simulink model "quantization3"  (Simulink 8.3)
settings: Solver=ode45  StartTime=0.0  StopTime=20  RelTol=1e-3
libraries: simulink x2
settings Model: Creator=Liu Guopin  LastModifiedBy=Liu Guopin
settings OptimizationCC: ExpressionDepthLimit=2147483647
settings DebuggingCC: FcnCallInpInsideContextMsg=UseLocalSettings  StrictBusMsg=Warning

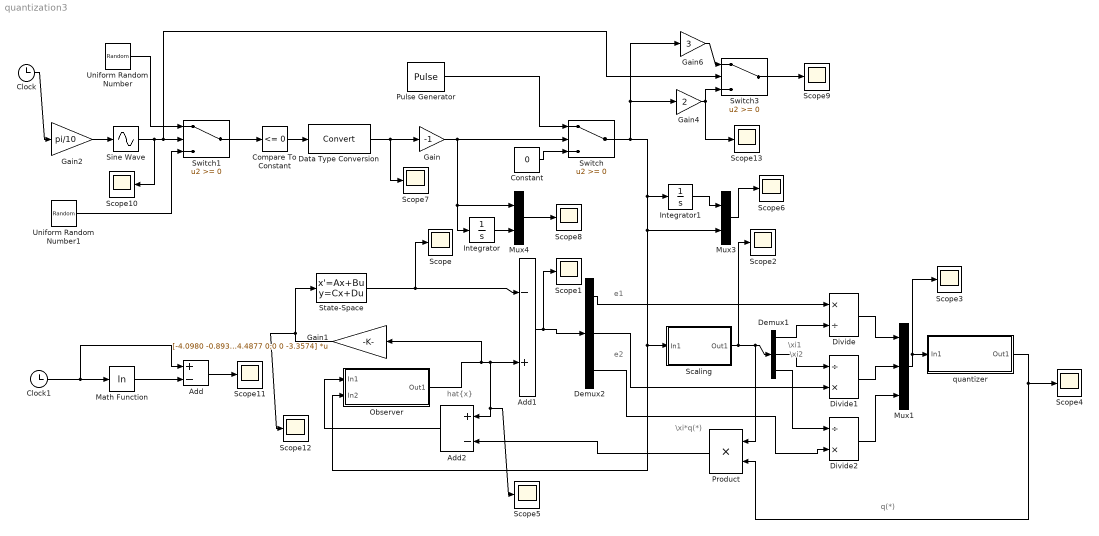
== system quantization3 ==
  note: e1
  note: e2
  note: \xi1
  note: \xi2
  note: hat{x}
  note: q(*)
  note: \xi*q(*)
  Add : Sum  Inputs=+-
  Add1 : Sum  Inputs=-+
  Add2 : Sum  Inputs=+-
  Clock : Clock
  Clock1 : Clock
  Compare To Constant : simulink/Logic and Bit Operations/Compare To Constant  relop=<=  const=0  OutDataTypeStr=boolean
  Constant : Constant  Value=0
  Data Type Conversion : DataTypeConversion
  Demux1 : Demux  Outputs=3
  Demux2 : Demux  Outputs=3
  Divide : Product  Inputs=*/
  Divide1 : Product  Inputs=/*
  Divide2 : Product  Inputs=/*
  Gain : Gain  Gain=-1
  Gain1 : Gain  Gain=[-4.0980 -0.8936 0; -0.8936 -4.4877 0;0 0 -3.3574]  Multiplication=Matrix(K*u) (u vector)
  Gain2 : Gain  Gain=pi/10
  Gain4 : Gain  Gain=2
  Gain6 : Gain  Gain=3
  Integrator : Integrator
  Integrator1 : Integrator
  Math Function : Math  Operator=log  SaturateOnIntegerOverflow=on
  Mux1 : Mux  Inputs=3
  Mux3 : Mux  Inputs=2
  Mux4 : Mux  Inputs=2
  Observer : Subsystem
  Product : Product  RndMeth=Zero
  Pulse Generator : DiscretePulseGenerator  PulseType=Time based  Period=0.1  PulseWidth=5
  Scaling : Subsystem
  Scope{,1..13} (14 alike) : Scope
      Scope1 settings: SaveName=ScopeData2
      Scope10 settings: SaveName=ScopeData11
      Scope11 settings: SaveName=ScopeData12
      Scope12 settings: SaveName=ScopeData15
      Scope13 settings: SaveName=ScopeData17
      Scope2 settings: SaveName=ScopeData3
      Scope3 settings: SaveName=ScopeData4
      Scope4 settings: SaveName=ScopeData5
      Scope5 settings: SaveName=ScopeData6
      Scope6 settings: SaveName=ScopeData7
      Scope7 settings: SaveName=ScopeData8
      Scope8 settings: SaveName=ScopeData9
      Scope9 settings: SaveName=ScopeData10
  Sine Wave : Sin  TimeSource=Use external signal  SampleTime=0
  State-Space : StateSpace  A=[2 1 0;0 2 0;0 0 1.5]  B=eye(3)  C=eye(3)  D=[0 0 0;0 0 0;0 0 0]  X0=[1.2;-0.8;0.5]
  Switch : Switch
  Switch1 : Switch
  Switch3 : Switch
  Uniform Random Number : UniformRandomNumber  Minimum=-1.37  Maximum=0.63  SampleTime=0.2
  Uniform Random Number1 : UniformRandomNumber  Minimum=-0.8  Maximum=1.2  SampleTime=0.2
  quantizer : Subsystem
  wires:
  Compare To Constant/1 -> Data Type Conversion/1
  Gain/1 -> Switch/2, Integrator/1, Mux4/1
  Data Type Conversion/1 -> Scope7/1, Gain/1
  State-Space/1 -> Add1/1, Scope/1
  Observer/1(Out1) -> Gain1/1, Add1/2, Add2/1, Scope5/1
  Gain1/1 -> State-Space/1, Scope12/1
  Scaling/1(Out1) -> Demux1/1, Product/1, Scope2/1
  Demux1/2 -> Divide1/1
  Demux1/1 -> Divide/2
  Demux2/1 -> Divide/1
  Demux2/2 -> Divide1/2
  Divide/1 -> Mux1/1
  Divide1/1 -> Mux1/2
  Mux1/1 -> quantizer/1(In1), Scope3/1
  quantizer/1(Out1) -> Product/2, Scope4/1
  Product/1 -> Add2/2
  Add2/1 -> Observer/1(In1)
  Constant/1 -> Switch/3
  Pulse Generator/1 -> Switch/1
  Switch/1 -> Integrator1/1, Scaling/1(In1), Observer/2(In2), Mux3/2, Gain6/1, Gain4/1
  Add1/1 -> Demux2/1, Scope1/1
  Clock/1 -> Gain2/1
  Gain2/1 -> Sine Wave/1
  Integrator1/1 -> Mux3/1
  Mux3/1 -> Scope6/1
  Integrator/1 -> Mux4/2
  Mux4/1 -> Scope8/1
  Sine Wave/1 -> Scope10/1, Switch1/2, Switch3/2
  Uniform Random Number1/1 -> Switch1/3
  Uniform Random Number/1 -> Switch1/1
  Switch1/1 -> Compare To Constant/1
  Clock1/1 -> Math Function/1, Add/1
  Math Function/1 -> Add/2
  Add/1 -> Scope11/1
  Demux1/3 -> Divide2/1
  Demux2/3 -> Divide2/2
  Divide2/1 -> Mux1/3
  Gain6/1 -> Switch3/1
  Gain4/1 -> Switch3/3, Scope13/1
  Switch3/1 -> Scope9/1

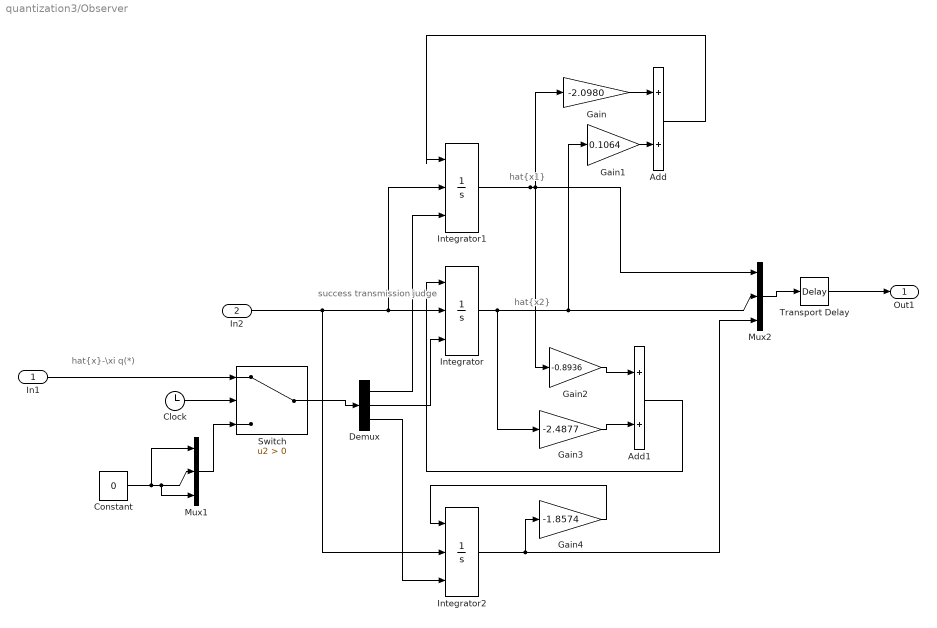
== system quantization3/Observer ==
  note: hat{x2}
  note: hat{x}-\xi q(*)
  note: success transmission judge
  note: hat{x1}
  In1 : Inport
  In2 : Inport  Port=2
  Add : Sum
  Add1 : Sum
  Clock : Clock
  Constant : Constant  Value=0
  Demux : Demux  Outputs=3
  Gain : Gain  Gain=-2.0980
  Gain1 : Gain  Gain=0.1064
  Gain2 : Gain  Gain=-0.8936
  Gain3 : Gain  Gain=-2.4877
  Gain4 : Gain  Gain=-1.8574
  Integrator : Integrator  ExternalReset=rising  InitialConditionSource=external
  Integrator1 : Integrator  ExternalReset=rising  InitialConditionSource=external
  Integrator2 : Integrator  ExternalReset=rising  InitialConditionSource=external
  Mux1 : Mux  Inputs=3
  Mux2 : Mux  Inputs=3
  Switch : Switch  Criteria=u2 > Threshold
  Transport Delay : TransportDelay  DelayTime=0.00000001
  Out1 : Outport
  wires:
  In1/1 -> Switch/1
  Clock/1 -> Switch/2
  Constant/1 -> Mux1/1, Mux1/2, Mux1/3
  Mux1/1 -> Switch/3
  Switch/1 -> Demux/1
  In2/1 -> Integrator/2, Integrator1/2, Integrator2/2
  Integrator/1 -> Mux2/2, Gain1/1, Gain3/1
  Demux/1 -> Integrator1/3
  Demux/2 -> Integrator/3
  Integrator1/1 -> Mux2/1, Gain/1, Gain2/1
  Gain1/1 -> Add/2
  Gain/1 -> Add/1
  Gain3/1 -> Add1/2
  Gain2/1 -> Add1/1
  Add/1 -> Integrator1/1
  Add1/1 -> Integrator/1
  Transport Delay/1 -> Out1/1
  Demux/3 -> Integrator2/3
  Mux2/1 -> Transport Delay/1
  Integrator2/1 -> Mux2/3, Gain4/1
  Gain4/1 -> Integrator2/1

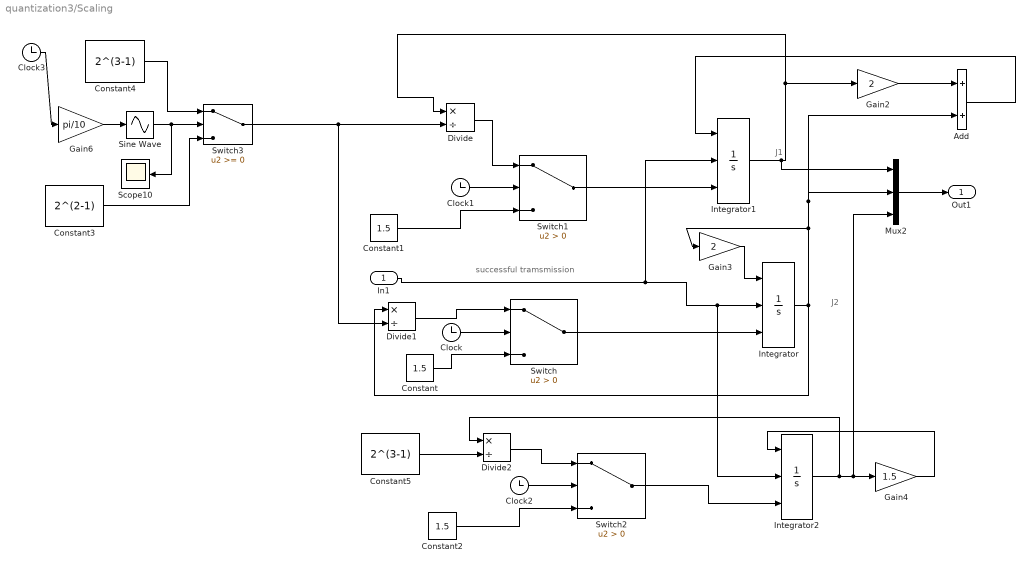
== system quantization3/Scaling ==
  note: J1
  note: J2
  note: successful tramsmission
  In1 : Inport
  Add : Sum
  Clock{,1..3} (4 alike) : Clock
  Constant : Constant  Value=1.5
  Constant1 : Constant  Value=1.5
  Constant2 : Constant  Value=1.5
  Constant3 : Constant  Value=2^(2-1)
  Constant4 : Constant  Value=2^(3-1)
  Constant5 : Constant  Value=2^(3-1)
  Divide : Product  Inputs=*/
  Divide1 : Product  Inputs=*/
  Divide2 : Product  Inputs=*/
  Gain2 : Gain  Gain=2
  Gain3 : Gain  Gain=2
  Gain4 : Gain  Gain=1.5
  Gain6 : Gain  Gain=pi/10
  Integrator : Integrator  ExternalReset=rising  InitialConditionSource=external
  Integrator1 : Integrator  ExternalReset=rising  InitialConditionSource=external
  Integrator2 : Integrator  ExternalReset=rising  InitialConditionSource=external
  Mux2 : Mux  Inputs=3
  Scope10 : Scope
      settings: SaveName=ScopeData14
  Sine Wave : Sin  TimeSource=Use external signal  SampleTime=0
  Switch : Switch  Criteria=u2 > Threshold
  Switch1 : Switch  Criteria=u2 > Threshold
  Switch2 : Switch  Criteria=u2 > Threshold
  Switch3 : Switch
  Out1 : Outport
  wires:
  Clock/1 -> Switch/2
  Constant/1 -> Switch/3
  Clock1/1 -> Switch1/2
  Constant1/1 -> Switch1/3
  Switch/1 -> Integrator/3
  Switch1/1 -> Integrator1/3
  In1/1 -> Integrator1/2, Integrator/2, Integrator2/2
  Integrator1/1 -> Gain2/1, Divide/1, Mux2/1
  Integrator/1 -> Add/2, Mux2/2, Gain3/1, Divide1/1
  Add/1 -> Integrator1/1
  Mux2/1 -> Out1/1
  Gain2/1 -> Add/1
  Gain3/1 -> Integrator/1
  Clock2/1 -> Switch2/2
  Constant2/1 -> Switch2/3
  Integrator2/1 -> Gain4/1, Mux2/3, Divide2/1
  Switch2/1 -> Integrator2/3
  Gain4/1 -> Integrator2/1
  Divide2/1 -> Switch2/1
  Clock3/1 -> Gain6/1
  Gain6/1 -> Sine Wave/1
  Sine Wave/1 -> Switch3/2, Scope10/1
  Constant3/1 -> Switch3/3
  Constant4/1 -> Switch3/1
  Divide/1 -> Switch1/1
  Switch3/1 -> Divide/2, Divide1/2
  Divide1/1 -> Switch/1
  Constant5/1 -> Divide2/2

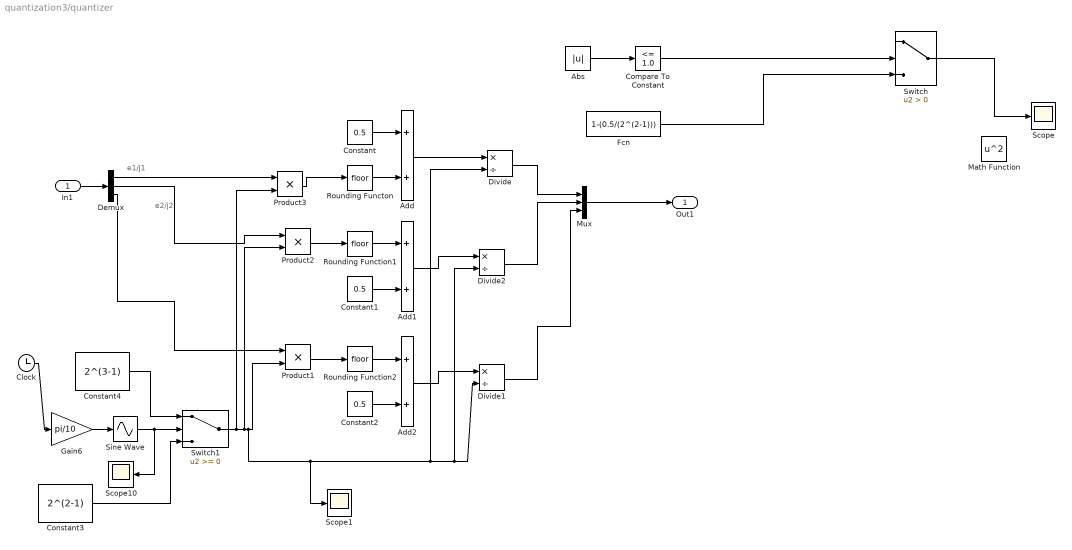
== system quantization3/quantizer ==
  note: e1/j1
  note: e2/j2
  In1 : Inport
  Abs : Abs
  Add : Sum
  Add1 : Sum
  Add2 : Sum
  Clock : Clock
  Compare To Constant : simulink/Logic and Bit Operations/Compare To Constant  SystemSampleTime=-1  relop=<=  const=1.0  LogicOutDataTypeMode=uint8  ZeroCross=off
  Constant : Constant  Value=0.5
  Constant1 : Constant  Value=0.5
  Constant2 : Constant  Value=0.5
  Constant3 : Constant  Value=2^(2-1)
  Constant4 : Constant  Value=2^(3-1)
  Demux : Demux  Outputs=3
  Divide : Product  Inputs=*/
  Divide1 : Product  Inputs=*/
  Divide2 : Product  Inputs=*/
  Fcn : Fcn  Expr=1-(0.5/(2^(2-1)))
  Gain6 : Gain  Gain=pi/10
  Math Function : Math  Operator=square  SaturateOnIntegerOverflow=on
  Mux : Mux  Inputs=3
  Product1 : Product  RndMeth=Zero
  Product2 : Product  RndMeth=Zero
  Product3 : Product  RndMeth=Zero
  Rounding Function1 : Rounding
  Rounding Function2 : Rounding
  Rounding Functon : Rounding
  Scope : Scope
  Scope1 : Scope
      settings: SaveName=ScopeData16
  Scope10 : Scope
      settings: SaveName=ScopeData13
  Sine Wave : Sin  TimeSource=Use external signal  SampleTime=0
  Switch : Switch  Criteria=u2 > Threshold
  Switch1 : Switch
  Out1 : Outport
  wires:
  In1/1 -> Demux/1
  Demux/1 -> Product3/1
  Abs/1 -> Compare To Constant/1
  Compare To Constant/1 -> Switch/2
  Rounding Functon/1 -> Add/2
  Fcn/1 -> Switch/3
  Demux/2 -> Product2/1
  Constant/1 -> Add/1
  Rounding Function1/1 -> Add1/1
  Constant1/1 -> Add1/2
  Product2/1 -> Rounding Function1/1
  Product3/1 -> Rounding Functon/1
  Add1/1 -> Divide2/1
  Switch/1 -> Scope/1
  Mux/1 -> Out1/1
  Add/1 -> Divide/1
  Divide/1 -> Mux/1
  Divide2/1 -> Mux/2
  Demux/3 -> Product1/1
  Rounding Function2/1 -> Add2/1
  Constant2/1 -> Add2/2
  Product1/1 -> Rounding Function2/1
  Add2/1 -> Divide1/1
  Divide1/1 -> Mux/3
  Clock/1 -> Gain6/1
  Gain6/1 -> Sine Wave/1
  Sine Wave/1 -> Switch1/2, Scope10/1
  Constant3/1 -> Switch1/3
  Constant4/1 -> Switch1/1
  Switch1/1 -> Product2/2, Product1/2, Divide1/2, Divide2/2, Divide/2, Scope1/1, Product3/2
